simulink model "comprehensive_model_with_rocks_trial"  (R2019a)
settings: Solver=FixedStepAuto  StartTime=0.0  StopTime=15  FixedStep=0.001  RelTol=1e-3
PreLoadFcn:
  | load('tumbleweed_constants.mat')
values from neighbouring files (symbols this model uses):
  Ar = 0.785398163397    [tumbleweed_constants.mat]
  CD = 0.8    [tumbleweed_constants.mat]
  d = 0.65    [tumbleweed_constants.mat]
  g = 9.81    [tumbleweed_constants.mat]
  Ixx = 1.29    [tumbleweed_constants.mat]
  Iyy = 1.29    [tumbleweed_constants.mat]
  Izz = 1.29    [tumbleweed_constants.mat]
  m = 1    [tumbleweed_constants.mat]
  maxr = 0.45    [tumbleweed_constants.mat]
  mf = 14    [tumbleweed_constants.mat]
  minr = 0.2    [tumbleweed_constants.mat]
  mu0 = 0.02    [tumbleweed_constants.mat]
  muk = 0.5    [tumbleweed_constants.mat]
  must = 0.8    [tumbleweed_constants.mat]
  R = cylR*ones(size(Theta,1),size(Theta,2))    [d3_animate.m]    (also in tumbleweed_constants.mat = 0.5)
  rest_coeff = 0.6    [tumbleweed_constants.mat]
  rho = 1.2    [tumbleweed_constants.mat]
  ts = 0.5    [tumbleweed_constants.mat]
  v_thres = 0.0001    [tumbleweed_constants.mat]
  vmax = 0.2    [tumbleweed_constants.mat]
  YY = 50    [tumbleweed_constants.mat]
libraries: simulink x2
(part 3 of 9)

== matlab function comprehensive_model_with_rocks_trial/bouncing_model1/only_bounce/MATLAB Function1 ==
  data: t input; states input; constraint_flag output; r_AO output; par_diffs output; rock_cents input; rock_radi input; jAp input; surf_num input; R parameter; surf_numch output
function [constraint_flag, r_AO, par_diffs, surf_numch] = surf_constraint_check(t, states, rock_cents, rock_radi, jAp, surf_num, R)
if t == 3.431
    disp(t);
end
surf_numch = surf_num;
r_TO = [states(7);states(8);states(9)];
O_v_TO =[states(4);states(5);states(6)];
%change the surface equation in the dist_calc function and par_diffs_calc
point_on_surf = [0;0];
smallest_dist = 0;
rock_radi = rock_radi';
if t== 2.922
    disp(states)
end
[point_on_surf, smallest_dist] = dist_calc(r_TO);
z_c = surf_eq(point_on_surf(1),point_on_surf(2),r_TO);
r_AO = [point_on_surf;z_c];
par_diffs = par_diffs_calc(r_AO);
        fx = par_diffs(1,1); 
        fy = par_diffs(2,1);
        fz = par_diffs(3,1);
        kO = [0;0;1];
        iO = [1;0;0];
        jO = [0;1;0];

        if(abs(fx)<=1e-10 && abs(fy)<=1e-10)
            kA = kO;
            jA = jO;
            iA = iO;
            O_c_A = eye(3);
            A_c_O = eye(3);
            flag = 1;
        else
        kA = [fx;fy;fz]/norm([fx;fy;fz]);
        jA = cross(kO,kA)/norm(cross(kO,kA));
        flag = 1;
        if((jAp.')*(jA) < 0)
            jA = -jA;
            flag = 2;
        end
        iA = cross(jA,kA);
        A_c_O = [iA'*iO, iA'*jO, iA'*kO; jA'*iO, jA'*jO, jA'*kO; kA'*iO, kA'*jO, kA'*kO];
        O_c_A = transpose(A_c_O);
        end
O_v_TOa = A_c_O*O_v_TO;  

if norm(r_AO - r_TO) <= R + 0.00005 && O_v_TOa(3) <= 0
    constraint_flag = 1;
elseif norm(r_AO - r_TO) <= R - 0.002 && O_v_TOa(3) <= 0
    constraint_flag = 1;    
else 
    constraint_flag = 0;
end
rock_coll_flag = 0;
rock_ind = 0;

for i = 1:size(rock_cents,2) 
    if norm(r_TO - rock_cents(:,i)) <= rock_radi(1,i) + R + 0.001
        kR = (r_TO - rock_cents(:,i))/norm(r_TO -  rock_cents(:,i));   
       if(abs(kR(1))<=1e-10 && abs(kR(2))<=1e-10)
            kR = kO;
            jR = jO;
            iR = iO;
            O_c_R = eye(3);
            R_c_O = eye(3);
            flag = 1;
       else
        jR = cross(kO,kR)/norm(cross(kO,kR));
        flag = 1;
        if((jAp.')*(jR) < 0)
            jR = -jR;
            flag = 2;
        end
        iR = cross(jR,kR);
        R_c_O = [iR'*iO, iR'*jO, iR'*kO; jR'*iO, jR'*jO, jR'*kO; kR'*iO, kR'*jO, kR'*kO];
        O_c_R = transpose(R_c_O);
        end
    O_v_TOr = R_c_O*O_v_TO;  
        if O_v_TOr(3)<= 0
            rock_coll_flag = 1;
            rock_ind = i;
        end
    end
end
if (rock_coll_flag == 1 && constraint_flag == 0) 
kR = (r_TO - rock_cents(:,rock_ind))/norm(r_TO -  rock_cents(:,rock_ind));
point_on_rock = rock_cents(:,rock_ind) + rock_radi(1,rock_ind)*kR;
r_AO = point_on_rock;
par_diffs = rock_pardiffs_calc(point_on_rock, rock_cents(:,rock_ind));
surf_numch = rock_ind;
constraint_flag = 1;
elseif (rock_coll_flag == 1 && constraint_flag == 1)
kR = (r_TO - rock_cents(:,rock_ind))/norm(r_TO -  rock_cents(:,rock_ind));
point_on_rock = rock_cents(:,rock_ind) + rock_radi(1,rock_ind)*kR;
r_AO = point_on_rock;
par_diffs = rock_pardiffs_calc(point_on_rock, rock_cents(:,rock_ind));
surf_numch = 0;
elseif (rock_coll_flag == 0 && constraint_flag == 1)
    surf_numch = 0;
end
end




function rock_pardiffs = rock_pardiffs_calc(point_on_rock, rock_center)
r_RO = point_on_rock; x_c = r_RO(1); y_c = r_RO(2); z_c = r_RO(3);
r_CO = rock_center;
fx = 2*(x_c - r_CO(1,1));
fy = 2*(y_c - r_CO(2,1));
fz = 2*(z_c - r_CO(3,1));
fxx = 2;
fxy = 0;
fxz = 0;
fyy = 2;
fyz = 0;
fzz = 2;
fxxx = 0;
fxxy = 0;
fxxz = 0;
fxyy = 0;
fxyz = 0;
fxzz = 0;
fyyy = 0;
fyyz = 0;
fyzz = 0;
fzzz = 0;
rock_pardiffs = [fx;fy;fz;fxx;fxy;fxz;fyy;fyz;fzz;fxxx;fxxy;fxxz;fxyy;fxyz;fxzz;fyyy;fyyz;fyzz;fzzz];
end



function z_c = surf_eq(x_c, y_c, r_TO)
% if r_TO(3) >= 0
%     if x_c^2 - 2*y_c < 0
%         z_c = 0;
%     else
%     z_c = sqrt(x_c^2 - 2*y_c);
%     end
% else
%     if x_c^2 - 2*y_c < 0
%         z_c = 0;
%     else
%     z_c = -sqrt(x_c^2 - 2*y_c);
%     end
% end
z_c = 0;%(4*exp(-((x_c-5)^2 + (y_c)^2)/(6^2))-6*exp(-((x_c-5)^2 + (y_c)^2)/(4^2)));%(-1*exp(-((x_c - 10)^2 + (y_c - 10)^2)/2^2) -5*exp(-((x_c - 10)^2 + (y_c - 15)^2)/5^2) + 5*exp(-((x_c - 10)^2 + (y_c + 10)^2)/5^2) - 3*exp(-((x_c - 20)^2 + (y_c +5)^2)/4^2) - 5*exp(-((x_c - 40)^2 + (y_c -10)^2)/6^2));
end

function par_diffs = par_diffs_calc(r_AO)

x_c = r_AO(1);
y_c = r_AO(2);
z_c = r_AO(3);

fx = 0;%4*exp(- (x_c - 5)^2/36 - y_c^2/36)*(x_c/18 - 5/18) - 6*exp(- (x_c - 5)^2/16 - y_c^2/16)*(x_c/8 - 5/8);
fy = 0;%(2*y_c*exp(- (x_c - 5)^2/36 - y_c^2/36))/9 - (3*y_c*exp(- (x_c - 5)^2/16 - y_c^2/16))/4;
fz = 1;
fxx = 0;%(2*exp(- (x_c - 5)^2/36 - y_c^2/36))/9 - (3*exp(- (x_c - 5)^2/16 - y_c^2/16))/4 + 6*exp(- (x_c - 5)^2/16 - y_c^2/16)*(x_c/8 - 5/8)^2 - 4*exp(- (x_c - 5)^2/36 - y_c^2/36)*(x_c/18 - 5/18)^2;
fxy = 0;%(3*y_c*exp(- (x_c - 5)^2/16 - y_c^2/16)*(x_c/8 - 5/8))/4 - (2*y_c*exp(- (x_c - 5)^2/36 - y_c^2/36)*(x_c/18 - 5/18))/9;
fxz = 0;
fyy = 0;%(2*exp(- (x_c - 5)^2/36 - y_c^2/36))/9 - (3*exp(- (x_c - 5)^2/16 - y_c^2/16))/4 + (3*y_c^2*exp(- (x_c - 5)^2/16 - y_c^2/16))/32 - (y_c^2*exp(- (x_c - 5)^2/36 - y_c^2/36))/81;
fyz = 0;
fzz = 0;
fxxx = 0;%(3*exp(- (x_c - 5)^2/16 - y_c^2/16)*(x_c/8 - 5/8))/4 + 6*exp(- (x_c - 5)^2/16 - y_c^2/16)*(x_c/32 - 5/32) - (2*exp(- (x_c - 5)^2/36 - y_c^2/36)*(x_c/18 - 5/18))/9 - 4*exp(- (x_c - 5)^2/36 - y_c^2/36)*(x_c/162 - 5/162) - 6*exp(- (x_c - 5)^2/16 - y_c^2/16)*(x_c/8 - 5/8)^3 + 4*exp(- (x_c - 5)^2/36 - y_c^2/36)*(x_c/18 - 5/18)^3;
fxxy = 0;%(3*y_c*exp(- (x_c - 5)^2/16 - y_c^2/16))/32 - (y_c*exp(- (x_c - 5)^2/36 - y_c^2/36))/81 - (3*y_c*exp(- (x_c - 5)^2/16 - y_c^2/16)*(x_c/8 - 5/8)^2)/4 + (2*y_c*exp(- (x_c - 5)^2/36 - y_c^2/36)*(x_c/18 - 5/18)^2)/9;
fxxz = 0;
fxyy = 0;%(3*exp(- (x_c - 5)^2/16 - y_c^2/16)*(x_c/8 - 5/8))/4 - (2*exp(- (x_c - 5)^2/36 - y_c^2/36)*(x_c/18 - 5/18))/9 - (3*y_c^2*exp(- (x_c - 5)^2/16 - y_c^2/16)*(x_c/8 - 5/8))/32 + (y_c^2*exp(- (x_c - 5)^2/36 - y_c^2/36)*(x_c/18 - 5/18))/81;
fxyz = 0;
fxzz = 0;
fyyy = 0;%(9*y_c*exp(- (x_c - 5)^2/16 - y_c^2/16))/32 - (y_c*exp(- (x_c - 5)^2/36 - y_c^2/36))/27 - (3*y_c^3*exp(- (x_c - 5)^2/16 - y_c^2/16))/256 + (y_c^3*exp(- (x_c - 5)^2/36 - y_c^2/36))/1458;
fyyz = 0;
fyzz = 0;
fzzz = 0;


% fx = -x_c;
% fy = 1;
% fz = z_c;
% fxx = -1;
% fxy = 0;
% fxz = 0;
% fyy = 0;
% fyz = 0;
% fzz = 1;
% fxxx = 0;
% fxxy = 0;
% fxxz = 0;
% fxyy = 0;
% fxyz = 0;
% fxzz = 0;
% fyyy = 0;
% fyyz = 0;
% fyzz = 0;
% fzzz = 0;
% 


par_diffs = [fx;fy;fz;fxx;fxy;fxz;fyy;fyz;fzz;fxxx;fxxy;fxxz;fxyy;fxyz;fxzz;fyyy;fyyz;fyzz;fzzz];
end

== matlab function comprehensive_model_with_rocks_trial/Subsystem1/MATLAB Function ==
  data: t input; y output size=3; ydot output size=3; states input; hit input; hit output; R parameter; y_new input; y_new output; err input; cum_err input; err output; cum_err output; rand_num input; stop_flag output
function [y, ydot,hit, y_new,err,cum_err,stop_flag] = reference_trajectory_generator(t,states,hit,R,y_new,err,cum_err,rand_num)

% xr = y_new;
% yr = 30*sin(xr/(30*pi));
% zr = R;
% 
% if abs(states(7) - xr) <= 0.5    
% xr = xr + 5;
% y_new = xr;
% cum_err = cum_err + abs(states(8) - yr);
% err = abs(states(8) - yr);
% yr = 30*sin(xr/(30*pi));
% zr = R; 
% end
% 
% xr_dot = 0;
% yr_dot = 0;
% zr_dot = 0;

if hit == 0
 xr = 800;
 yr = 1000;
 zr = R;
        
 
xr_dot = 0;
yr_dot = 0;
zr_dot = 0;
elseif hit == 1
 xr = states(7);
 yr = y_new(2);
 zr = R;
        
 
xr_dot = 0;
yr_dot = 0;
zr_dot = 0;
% elseif hit == 2
%      xr = 150;
%  yr = -40;
%  zr = R;
%         
% % 
% xr_dot = 0;
% yr_dot = 0;
% zr_dot = 0;
% elseif hit == 3
% xr = 200;
%  yr = -10;
%  zr = R;
%         
% 
% xr_dot = 0;
% yr_dot = 0;
% zr_dot = 0;
else
 xr = states(7);
 yr = y_new(2);
 zr = R;


xr_dot = 0;
yr_dot = 0;
zr_dot = 0;
end
% 
if hit == 0 && abs(states(7) - xr )<=0.5
    hit = 1;
    y_new = [states(7);states(8)];
% elseif hit == 1 && abs(states(7) -xr)<=0.5
%     hit = 2;
% elseif hit == 2 && abs(states(8) - yr)<=0.5
%     hit = 3;
% elseif hit == 3 && abs(states(8) - yr)<=0.5
%     hit = 4;
else
    hit = hit;
end
% 
% xr = 0.1*t;
% yr = 15*sin(0.1/4*t);
% zr = R;
% 
% xr_dot = 0.1;
% yr_dot = 15*cos(0.1/4*t)*(0.1/4);
% zr_dot = 0;
% if abs(xr - 10) <= 0.5
%     xr = states(7);
%     yr = 1000;
%     zr = R;
% else
% xr = states(7);
% yr = 1000;
% zr = R;
% end
% 
% xr_dot = 0;
% yr_dot = 0;
% zr_dot =0;
% xr = 30*cos(0.062/3*t);
% yr = 30*sin(0.062/3*t);
% zr = R;
% xr_dot = -30*sin(0.062/3*t)*(0.062/3);
% yr_dot = 30*cos(0.062/3*t)*(0.062/3);
% zr_dot = 0;

% 
% if abs(states(7) - y_new(1))<=0.5
% cum_err = abs(states(8) - y_new(2));
% y_new(1) = y_new(1) + 50;    
% if mod(((states(7) - rem(states(7),500))/500),2) == 0 
% y_new(2) = states(8) + 15*rand_num;
% else
%     y_new(2) = states(8) - 15*rand_num;
% end
% err = [states(7);states(8)];
% 
% 
% end
% xr = y_new(1);
% yr = y_new(2);
% zr = R;
% 
% xr_dot = 0;
% yr_dot = 0;
% zr_dot = 0;

if abs(states(7) - y_new(1))<=1
    y_new(1) = y_new(1) + 10;   
    y_new(2) = 50*sin(y_new(1)*2*pi/750);
    err = [states(7);states(8)];
end

xr = y_new(1);
yr = y_new(2);
zr = R;
xr_dot = 0;
yr_dot = 0;
zr_dot = 0;

if states(7) > 750
    stop_flag = 1;
else
    stop_flag = 0;
end
y = [xr;yr;zr];
ydot = [xr_dot; yr_dot; zr_dot];
 

end

== matlab function comprehensive_model_with_rocks_trial/command filter based backstepper/Subsystem1/MATLAB Function ==
  data: u input; f3_u output size=3; u_dot input; u_ddot input; states input; FW input; v_thres parameter; d parameter; R parameter; mu0 parameter; mf parameter; m parameter; Izz parameter; Iyy parameter; Ixx parameter; g parameter
function f3_u = f3u_calculator(u,u_dot,u_ddot,states,FW,v_thres, d, R, mu0, mf, m, Izz, Iyy, Ixx, g)
I_T = [Ixx,0,0;0,Iyy,0;0,0,Izz];
r_m1T = [u(1);0;0];             T_v_m1T = [u_dot(1);0;0]; T_a_m1T = [u_ddot(1);0;0];
r_m2T = [-(d - u(1));0;0];      T_v_m2T = [u_dot(1);0;0]; T_a_m2T = [u_ddot(1);0;0];
r_m3T = [0;u(2);0];             T_v_m3T = [0;u_dot(2);0]; T_a_m3T = [0;u_ddot(2);0];
r_m4T = [0;-(d - u(2));0];      T_v_m4T = [0;u_dot(2);0]; T_a_m4T = [0;u_ddot(2);0];
r_m5T = [0;0;u(3)];             T_v_m5T = [0;0;u_dot(3)]; T_a_m5T = [0;0;u_ddot(3)];
r_m6T = [0;0;-(d - u(3))];      T_v_m6T = [0;0;u_dot(3)]; T_a_m6T = [0;0;u_ddot(3)];
r_CMT = m*(r_m1T + r_m2T + r_m3T + r_m4T + r_m5T + r_m6T)/(6*m+mf);
T_v_CMT = m*(T_v_m1T + T_v_m2T + T_v_m3T + T_v_m4T + T_v_m5T + T_v_m6T)/(6*m+mf);
T_a_CMT = m*(T_a_m1T + T_a_m2T + T_a_m3T + T_a_m4T + T_a_m5T + T_a_m6T)/(6*m+mf);
r_CMTx = Vx(r_CMT);r_m1Tx = Vx(r_m1T);r_m2Tx = Vx(r_m2T);r_m3Tx = Vx(r_m3T);
r_m4Tx = Vx(r_m4T);r_m5Tx = Vx(r_m5T);r_m6Tx = Vx(r_m6T);
q0 = states(10);q1=states(11);q2=states(12);q3=states(13);
T_c_O = [q0^2 + q1^2 - q2^2 - q3^2, 2*(q1*q2 + q0*q3), 2*(q1*q3 - q0*q2);...
       2*(q1*q2 - q0*q3), q0^2 - q1^2 + q2^2 - q3^2, 2*(q2*q3 + q0*q1);...
       2*(q1*q3 + q0*q2), 2*(q2*q3 - q0*q1), q0^2 - q1^2 - q2^2 + q3^2];
O_c_T = transpose(T_c_O);  
r_PT = [0;0;-R];
r_PTx = Vx([0;0;-R]);
O_w_T = [states(1);states(2);states(3)]; O_w_Tx =Vx(O_w_T);

O_vel_TO = Vx(O_c_T*O_w_T)*[0;0;R];
u_TO = O_vel_TO(1);
v_TO = O_vel_TO(2);

murr = mu0*tanh((u_TO^2 + v_TO^2)/v_thres); 
roll_rest_coeff = [1,0,-murr*u_TO/sqrt(u_TO^2 + v_TO^2);0,1,-murr*v_TO/sqrt(u_TO^2 + v_TO^2);0,0,1];
FG = [0;0;-(mf+6*m)*g];
FR  = -murr*norm(FG)/sqrt(u_TO^2 + v_TO^2)*[u_TO; v_TO; 0];

f3_u = zeros(3,1);
Amat = I_T + (mf + 6*m)*r_CMTx*T_c_O*r_PTx*O_c_T - m*r_m1Tx*r_m1Tx - m*r_m2Tx*r_m2Tx...
       - m*r_m3Tx*r_m3Tx - m*r_m4Tx*r_m4Tx - m*r_m5Tx*r_m5Tx - m*r_m6Tx*r_m6Tx...
       - (mf + 6*m)*Vx(T_c_O*r_PT)*Vx(T_c_O*r_PT) + (mf + 6*m)*Vx(T_c_O*r_PT)*r_CMTx;
  %some mistakes here. check again 
Bvec = -cross(O_w_T,I_T*O_w_T) - m*cross(r_m1T,2*O_w_Tx*T_v_m1T + O_w_Tx*O_w_Tx*r_m1T)...
       - m*r_m2Tx*(T_a_m2T + 2*O_w_Tx*T_v_m2T + O_w_Tx*O_w_Tx*r_m2T)...
       - m*r_m3Tx*(T_a_m3T + 2*O_w_Tx*T_v_m3T + O_w_Tx*O_w_Tx*r_m3T)...
       - m*r_m4Tx*(T_a_m4T + 2*O_w_Tx*T_v_m4T + O_w_Tx*O_w_Tx*r_m4T)...
       - m*r_m5Tx*(T_a_m5T + 2*O_w_Tx*T_v_m5T + O_w_Tx*O_w_Tx*r_m5T)...
       - m*r_m6Tx*(T_a_m6T + 2*O_w_Tx*T_v_m6T + O_w_Tx*O_w_Tx*r_m6T)...
       + r_CMTx*T_c_O*FG + (mf + 6*m)*cross(T_c_O*r_PT, T_a_CMT + ...
         2*O_w_Tx*T_v_CMT + O_w_Tx*O_w_Tx*r_CMT) - T_c_O*cross(r_PT, FG) ...
         - T_c_O*cross(r_PT, FW);%- T_c_O*cross(r_PT, FR);
f3_u = inv(Amat)*Bvec;
end

== matlab function comprehensive_model_with_rocks_trial/bouncing_model/MATLAB Function ==
  data: t input; states_inair input; states output; states_onsurface input; FW_inair input; FW_onsurface input; inair_flag input; FW output; inactive_time input; inactive_time output; stop_flag output
function [states, FW, inactive_time, stop_flag] = merger(t,states_inair, states_onsurface, FW_inair, FW_onsurface, inair_flag, inactive_time)
if inair_flag > 0
    states = states_inair;
    FW = FW_inair;
    if norm(states) == 0
        states = states_onsurface;
        FW = FW_onsurface;
    end
else
    states = states_onsurface;
    FW = FW_onsurface;
    if norm(states) == 0
        states = states_inair;
         FW = FW_inair;
    end
    if mod(t,0.1) == 0
        if norm(states(4:6)) <= 0.005
            inactive_time = inactive_time + 0.1;
        else
            inactive_time = 0;
        end
    end
end

if inactive_time >= 50
    stop_flag = 1;
else
    stop_flag = 0;
end

end

== matlab function comprehensive_model_with_rocks_trial/bouncing_model/onsurface_model/MATLAB Function11 ==
  data: states input; wv input; FW output; CD parameter; rho parameter; Ar parameter
function FW = wind_force_calc(states,wv, CD, rho, Ar)
O_v_wO = [wv;0;0];
O_v_TO = [states(4);states(5);states(6)];
O_v_Tw = O_v_TO - O_v_wO;
FW = -0.5*CD*rho*Ar*norm(O_v_Tw)^2*O_v_Tw/norm(O_v_Tw);
%FW = zeros(3,1);
end

== matlab function comprehensive_model_with_rocks_trial/bouncing_model/onsurface_model/MATLAB Function2 ==
  data: r_AO input; r_AO0 input; roll_reset_flag input; par_diffs output; surf_num input; rock_cents input
function par_diffs = par_diffs_calc(r_AO, r_AO0, roll_reset_flag, surf_num, rock_cents)
if roll_reset_flag == 1
    r_AO = r_AO0;
end
x_c = r_AO(1);
y_c = r_AO(2);
z_c = r_AO(3);

if surf_num == 0
fx = 0;%4*exp(- (x_c - 5)^2/36 - y_c^2/36)*(x_c/18 - 5/18) - 6*exp(- (x_c - 5)^2/16 - y_c^2/16)*(x_c/8 - 5/8);
fy = 0;%(2*y_c*exp(- (x_c - 5)^2/36 - y_c^2/36))/9 - (3*y_c*exp(- (x_c - 5)^2/16 - y_c^2/16))/4;
fz = 1;
fxx = 0;%(2*exp(- (x_c - 5)^2/36 - y_c^2/36))/9 - (3*exp(- (x_c - 5)^2/16 - y_c^2/16))/4 + 6*exp(- (x_c - 5)^2/16 - y_c^2/16)*(x_c/8 - 5/8)^2 - 4*exp(- (x_c - 5)^2/36 - y_c^2/36)*(x_c/18 - 5/18)^2;
fxy = 0;%(3*y_c*exp(- (x_c - 5)^2/16 - y_c^2/16)*(x_c/8 - 5/8))/4 - (2*y_c*exp(- (x_c - 5)^2/36 - y_c^2/36)*(x_c/18 - 5/18))/9;
fxz = 0;
fyy = 0;%(2*exp(- (x_c - 5)^2/36 - y_c^2/36))/9 - (3*exp(- (x_c - 5)^2/16 - y_c^2/16))/4 + (3*y_c^2*exp(- (x_c - 5)^2/16 - y_c^2/16))/32 - (y_c^2*exp(- (x_c - 5)^2/36 - y_c^2/36))/81;
fyz = 0;
fzz = 0;
fxxx = 0;%(3*exp(- (x_c - 5)^2/16 - y_c^2/16)*(x_c/8 - 5/8))/4 + 6*exp(- (x_c - 5)^2/16 - y_c^2/16)*(x_c/32 - 5/32) - (2*exp(- (x_c - 5)^2/36 - y_c^2/36)*(x_c/18 - 5/18))/9 - 4*exp(- (x_c - 5)^2/36 - y_c^2/36)*(x_c/162 - 5/162) - 6*exp(- (x_c - 5)^2/16 - y_c^2/16)*(x_c/8 - 5/8)^3 + 4*exp(- (x_c - 5)^2/36 - y_c^2/36)*(x_c/18 - 5/18)^3;
fxxy = 0;%(3*y_c*exp(- (x_c - 5)^2/16 - y_c^2/16))/32 - (y_c*exp(- (x_c - 5)^2/36 - y_c^2/36))/81 - (3*y_c*exp(- (x_c - 5)^2/16 - y_c^2/16)*(x_c/8 - 5/8)^2)/4 + (2*y_c*exp(- (x_c - 5)^2/36 - y_c^2/36)*(x_c/18 - 5/18)^2)/9;
fxxz = 0;
fxyy = 0;%(3*exp(- (x_c - 5)^2/16 - y_c^2/16)*(x_c/8 - 5/8))/4 - (2*exp(- (x_c - 5)^2/36 - y_c^2/36)*(x_c/18 - 5/18))/9 - (3*y_c^2*exp(- (x_c - 5)^2/16 - y_c^2/16)*(x_c/8 - 5/8))/32 + (y_c^2*exp(- (x_c - 5)^2/36 - y_c^2/36)*(x_c/18 - 5/18))/81;
fxyz = 0;
fxzz = 0;
fyyy = 0;%(9*y_c*exp(- (x_c - 5)^2/16 - y_c^2/16))/32 - (y_c*exp(- (x_c - 5)^2/36 - y_c^2/36))/27 - (3*y_c^3*exp(- (x_c - 5)^2/16 - y_c^2/16))/256 + (y_c^3*exp(- (x_c - 5)^2/36 - y_c^2/36))/1458;
fyyz = 0;
fyzz = 0;
fzzz = 0;
else 

r_CO = rock_cents(:,surf_num).';
fx = 2*(x_c - r_CO(1));
fy = 2*(y_c - r_CO(2));
fz = 2*(z_c - r_CO(3));
fxx = 2;
fxy = 0;
fxz = 0;
fyy = 2;
fyz = 0;
fzz = 2;
fxxx = 0;
fxxy = 0;
fxxz = 0;
fxyy = 0;
fxyz = 0;
fxzz = 0;
fyyy = 0;
fyyz = 0;
fyzz = 0;
fzzz = 0;
end


% fx = -x_c;
% fy = 1;
% fz = z_c;
% fxx = -1;
% fxy = 0;
% fxz = 0;
% fyy = 0;
% fyz = 0;
% fzz = 1;
% fxxx = 0;
% fxxy = 0;
% fxxz = 0;
% fxyy = 0;
% fxyz = 0;
% fxzz = 0;
% fyyy = 0;
% fyyz = 0;
% fyzz = 0;
% fzzz = 0;
par_diffs = [fx;fy;fz;fxx;fxy;fxz;fyy;fyz;fzz;fxxx;fxxy;fxxz;fxyy;fxyz;fxzz;fyyy;fyyz;fyzz;fzzz];
end

== matlab function comprehensive_model_with_rocks_trial/bouncing_model/onsurface_model/MATLAB Function3 ==
  data: O_c_A input; states input; FN input; inair_flag output; FN output
function [inair_flag,FN] = inair_flag_set(O_c_A,states,FN)
O_v_TO = states(4:6,1);
A_c_O = O_c_A';
O_v_TOa = A_c_O*O_v_TO;
if FN < 0 || O_v_TOa(3) > 0.0001
    inair_flag = 1;
    FN = -1;
elseif O_v_TOa(3) < -0.008
    inair_flag = 1;
    FN = 100;
else
    inair_flag = 0;
end
end

== matlab function comprehensive_model_with_rocks_trial/bouncing_model/only_bounce/MATLAB Function2 ==
  data: t input; states input; u input; r_AO input; constraint_flag input; states output; roll_reset_flag output; FN input; inair_reset_flag output; par_diffs input; jAp input; surf_numch input; surf_nump input; rest_coeff parameter; m parameter; mf parameter; Ixx parameter; R parameter; jA output; must parameter; muk parameter; FN output; surf_num output; Iyy parameter; Izz parameter
function [states, roll_reset_flag, inair_reset_flag, jA, FN, surf_num] = collision_state_set(t,states, u,r_AO, constraint_flag, FN, par_diffs, jAp, surf_numch, surf_nump, rest_coeff, m, mf, Ixx, R, must, muk, Iyy, Izz)
%u1 u2 u3 u4 u5 u6 S1 S2 S3
surf_num = surf_nump;
roll_reset_flag = 0;
inair_reset_flag = 0;
O_w_T = [states(1);states(2);states(3)];
O_v_TO = [states(4);states(5);states(6)];
r_TO = [states(7);states(8);states(9)];
q = [states(10);states(11);states(12);states(13)];
q0 = q(1); q1 = q(2); q2 = q(3); q3 = q(4);

        fx = par_diffs(1,1); 
        fy = par_diffs(2,1);
        fz = par_diffs(3,1);
        kO = [0;0;1];
        iO = [1;0;0];
        jO = [0;1;0];

        if(abs(fx)<=1e-10 && abs(fy)<=1e-10)
            kA = kO;
            jA = jO;
            iA = iO;
            O_c_A = eye(3);
            A_c_O = eye(3);
            flag = 1;
        else
        kA = [fx;fy;fz]/norm([fx;fy;fz]);
        jA = cross(kO,kA)/norm(cross(kO,kA));
        flag = 1;
        if((jAp.')*(jA) < 0)
            jA = -jA;
            flag = 2;
        end
        iA = cross(jA,kA);
        A_c_O = [iA'*iO, iA'*jO, iA'*kO; jA'*iO, jA'*jO, jA'*kO; kA'*iO, kA'*jO, kA'*kO];
        O_c_A = transpose(A_c_O);
        end
O_v_TOa = A_c_O*O_v_TO;        
        
if mod(t,0.001) == 0
if constraint_flag == 0
    inair_flag = true;
 elseif constraint_flag == 1 && FN == 0
             inair_flag = false;
            roll_reset_flag = 1;
            r_TO = r_AO + R*kA;
            surf_num = surf_numch;
elseif constraint_flag == 1 && O_v_TOa(3) >= 0.0001
    inair_flag = true;    
else 
 %%collision response
     
        T_c_O = [q0^2 + q1^2 - q2^2 - q3^2, 2*(q1*q2 + q0*q3), 2*(q1*q3 - q0*q2);...
        2*(q1*q2 - q0*q3), q0^2 - q1^2 + q2^2 - q3^2, 2*(q2*q3 + q0*q1);...
        2*(q1*q3 + q0*q2), 2*(q2*q3 - q0*q1), q0^2 - q1^2 - q2^2 + q3^2];
        O_c_T = T_c_O.';
       
        
        
        T_c_A = T_c_O*O_c_A;
        A_c_T = T_c_A.';
        
        
        l1 = u(1); l2 = u(2); l3 = u(3); l4 = u(4); l5 = u(5); l6 = u(6);
        L33 = Ixx + m*(l3^2 + l4^2 + l5^2 + l6^2);
        L11 = Iyy + m*(l1^2 + l2^2 + l5^2 + l6^2);
        L22 = Izz + m*(l3^2 + l4^2 + l1^2 + l2^2);
        L = A_c_T*[L33,0,0;0,L11,0;0,0,L22]*T_c_A;
        L11 = L(2,2);
        L22 = L(3,3);
        L33 = L(1,1);
        
        mT = mf +6*m;

        w = A_c_T*(O_w_T);
        v = A_c_O*O_v_TO;

        u3 = w(1,1);
        u2 = w(3,1);
        u1 = w(2,1);

        u6 = v(1,1);
        u5 = v(3,1);
        u4 = v(2,1);


        u5_n = -rest_coeff*u5;  
        if abs(u5_n) <= 0.005 %&& FN > 0
            u5_n = 0;
            inair_flag = false;
            roll_reset_flag = 1;
            surf_num = surf_numch;
            r_TO = r_AO + R*kA;
%         elseif abs(u5_n) <= 0.005 && FN < 0
%             u5_n = 0;
%             inair_flag = true;
%             r_TO = r_AO + R*kA;   
        else
            inair_flag = true;
            inair_reset_flag = 1;
             r_TO = r_AO + R*kA;
             FN = 100;
        end
        u2_n = u2;
        u3_n = (L33*u3 - mT*R*u4)/(mT*R^2 + L33);
        u4_n = -R*u3_n;
        u1_n = (L11*u1 + mT*R*u6)/(mT*R^2 + L11);
        u6_n = R*u1_n;
        S1 = mT*(u4_n - u4);
        S2 = mT*(u5_n - u5);
        S3 = mT*(u6_n - u6);

        if ~(sqrt(S1^2 + S3^2) < must*norm(S2))
            alpha = u4 + R*u3;
            gamma = u6 - R*u1;
            k1 = 1/mT + R^2/L11;
            k3 = 1/mT + R^2/L33;
            
            if abs(alpha) > 0
                S1 = S1solve(S2, muk,alpha, gamma, k1, k3); 
                S3 = gamma*S1/(alpha + (k3 - k1)*S1);
                u1_n = u1 - R*S3/L11;
                u3_n = u3 + R*S1/L33;
                u4_n = u4 + S1/mT;
                u6_n = u6 + S3/mT;
            else 
                S3 = S1solve(S2, muk, gamma, alpha, k3, k1);
                S1 = alpha*S3/(gamma + (k1 - k3)*S3);
                u1_n = u1 - R*S3/L11;
                u3_n = u3 + R*S1/L33;
                u4_n = u4 + S1/mT;
                u6_n = u6 + S3/mT;
            end
            
        end

        O_w_T = T_c_A*[u3_n;u1_n;u2_n];
        O_v_TO = O_c_A*[u6_n; u4_n; u5_n];
end
else
    if  constraint_flag == 0
        inair_flag = true;
    else
        inair_flag = false;
    end
end

states = [O_w_T;O_v_TO;r_TO;q];
end

== matlab function comprehensive_model_with_rocks_trial/bouncing_model/only_bounce/MATLAB Function1 ==
  data: t input; states input; constraint_flag output; r_AO output; par_diffs output; rock_cents input; rock_radi input; jAp input; surf_num input; R parameter; surf_numch output
function [constraint_flag, r_AO, par_diffs, surf_numch] = surf_constraint_check(t, states, rock_cents, rock_radi, jAp, surf_num, R)
surf_numch = surf_num;
r_TO = [states(7);states(8);states(9)];
O_v_TO =[states(4);states(5);states(6)];
%change the surface equation in the dist_calc function and par_diffs_calc
point_on_surf = [0;0];
smallest_dist = 0;
rock_radi = rock_radi';
 [point_on_surf, smallest_dist] = dist_calc(r_TO);
% point_on_surf = [r_TO(1);r_TO(2)];
% smallest_dist = r_TO(3);
z_c = surf_eq(point_on_surf(1),point_on_surf(2),r_TO);
r_AO = [point_on_surf;z_c];
par_diffs = par_diffs_calc(r_AO);
        fx = par_diffs(1,1); 
        fy = par_diffs(2,1);
        fz = par_diffs(3,1);
        kO = [0;0;1];
        iO = [1;0;0];
        jO = [0;1;0];

        if(abs(fx)<=1e-10 && abs(fy)<=1e-10)
            kA = kO;
            jA = jO;
            iA = iO;
            O_c_A = eye(3);
            A_c_O = eye(3);
            flag = 1;
        else
        kA = [fx;fy;fz]/norm([fx;fy;fz]);
        jA = cross(kO,kA)/norm(cross(kO,kA));
        flag = 1;
        if((jAp.')*(jA) < 0)
            jA = -jA;
            flag = 2;
        end
        iA = cross(jA,kA);
        A_c_O = [iA'*iO, iA'*jO, iA'*kO; jA'*iO, jA'*jO, jA'*kO; kA'*iO, kA'*jO, kA'*kO];
        O_c_A = transpose(A_c_O);
        end
O_v_TOa = A_c_O*O_v_TO;  

if norm(r_AO - r_TO) <= R + 0.00005 && O_v_TOa(3) <= 0
    constraint_flag = 1;
elseif norm(r_AO - r_TO) <= R - 0.002 && O_v_TOa(3) <= 0
    constraint_flag = 1;    
else 
    constraint_flag = 0;
end
rock_coll_flag = 0;
rock_ind = 0;

for i = 1:size(rock_cents,2) 
    if norm(r_TO - rock_cents(:,i)) <= rock_radi(1,i) + R + 0.001
        kR = (r_TO - rock_cents(:,i))/norm(r_TO -  rock_cents(:,i));   
       if(abs(kR(1))<=1e-10 && abs(kR(2))<=1e-10)
            kR = kO;
            jR = jO;
            iR = iO;
            O_c_R = eye(3);
            R_c_O = eye(3);
            flag = 1;
       else
        jR = cross(kO,kR)/norm(cross(kO,kR));
        flag = 1;
        if((jAp.')*(jR) < 0)
            jR = -jR;
            flag = 2;
        end
        iR = cross(jR,kR);
        R_c_O = [iR'*iO, iR'*jO, iR'*kO; jR'*iO, jR'*jO, jR'*kO; kR'*iO, kR'*jO, kR'*kO];
        O_c_R = transpose(R_c_O);
        end
    O_v_TOr = R_c_O*O_v_TO;  
        if O_v_TOr(3)<= 0
            rock_coll_flag = 1;
            rock_ind = i;
        end
    end
end
if (rock_coll_flag == 1 && constraint_flag == 0) 
kR = (r_TO - rock_cents(:,rock_ind))/norm(r_TO -  rock_cents(:,rock_ind));
point_on_rock = rock_cents(:,rock_ind) + rock_radi(1,rock_ind)*kR;
r_AO = point_on_rock;
par_diffs = rock_pardiffs_calc(point_on_rock, rock_cents(:,rock_ind));
surf_numch = rock_ind;
constraint_flag = 1;
elseif (rock_coll_flag == 1 && constraint_flag == 1)
kR = (r_TO - rock_cents(:,rock_ind))/norm(r_TO -  rock_cents(:,rock_ind));
point_on_rock = rock_cents(:,rock_ind) + rock_radi(1,rock_ind)*kR;
r_AO = point_on_rock;
par_diffs = rock_pardiffs_calc(point_on_rock, rock_cents(:,rock_ind));
surf_numch = 0;
elseif (rock_coll_flag == 0 && constraint_flag == 1)
    surf_numch = 0;
end
end




function rock_pardiffs = rock_pardiffs_calc(point_on_rock, rock_center)
r_RO = point_on_rock; x_c = r_RO(1); y_c = r_RO(2); z_c = r_RO(3);
r_CO = rock_center;
fx = 2*(x_c - r_CO(1,1));
fy = 2*(y_c - r_CO(2,1));
fz = 2*(z_c - r_CO(3,1));
fxx = 2;
fxy = 0;
fxz = 0;
fyy = 2;
fyz = 0;
fzz = 2;
fxxx = 0;
fxxy = 0;
fxxz = 0;
fxyy = 0;
fxyz = 0;
fxzz = 0;
fyyy = 0;
fyyz = 0;
fyzz = 0;
fzzz = 0;
rock_pardiffs = [fx;fy;fz;fxx;fxy;fxz;fyy;fyz;fzz;fxxx;fxxy;fxxz;fxyy;fxyz;fxzz;fyyy;fyyz;fyzz;fzzz];
end



function z_c = surf_eq(x_c, y_c, r_TO)
% if r_TO(3) >= 0
%     if x_c^2 - 2*y_c < 0
%         z_c = 0;
%     else
%     z_c = sqrt(x_c^2 - 2*y_c);
%     end
% else
%     if x_c^2 - 2*y_c < 0
%         z_c = 0;
%     else
%     z_c = -sqrt(x_c^2 - 2*y_c);
%     end
% end
z_c = 0;%(4*exp(-((x_c-5)^2 + (y_c)^2)/(6^2))-6*exp(-((x_c-5)^2 + (y_c)^2)/(4^2)));%(-1*exp(-((x_c - 10)^2 + (y_c - 10)^2)/2^2) -5*exp(-((x_c - 10)^2 + (y_c - 15)^2)/5^2) + 5*exp(-((x_c - 10)^2 + (y_c + 10)^2)/5^2) - 3*exp(-((x_c - 20)^2 + (y_c +5)^2)/4^2) - 5*exp(-((x_c - 40)^2 + (y_c -10)^2)/6^2));
end

function par_diffs = par_diffs_calc(r_AO)

x_c = r_AO(1);
y_c = r_AO(2);
z_c = r_AO(3);

fx = 0;%4*exp(- (x_c - 5)^2/36 - y_c^2/36)*(x_c/18 - 5/18) - 6*exp(- (x_c - 5)^2/16 - y_c^2/16)*(x_c/8 - 5/8);
fy = 0;%(2*y_c*exp(- (x_c - 5)^2/36 - y_c^2/36))/9 - (3*y_c*exp(- (x_c - 5)^2/16 - y_c^2/16))/4;
fz = 1;
fxx = 0;%(2*exp(- (x_c - 5)^2/36 - y_c^2/36))/9 - (3*exp(- (x_c - 5)^2/16 - y_c^2/16))/4 + 6*exp(- (x_c - 5)^2/16 - y_c^2/16)*(x_c/8 - 5/8)^2 - 4*exp(- (x_c - 5)^2/36 - y_c^2/36)*(x_c/18 - 5/18)^2;
fxy = 0;%(3*y_c*exp(- (x_c - 5)^2/16 - y_c^2/16)*(x_c/8 - 5/8))/4 - (2*y_c*exp(- (x_c - 5)^2/36 - y_c^2/36)*(x_c/18 - 5/18))/9;
fxz = 0;
fyy = 0;%(2*exp(- (x_c - 5)^2/36 - y_c^2/36))/9 - (3*exp(- (x_c - 5)^2/16 - y_c^2/16))/4 + (3*y_c^2*exp(- (x_c - 5)^2/16 - y_c^2/16))/32 - (y_c^2*exp(- (x_c - 5)^2/36 - y_c^2/36))/81;
fyz = 0;
fzz = 0;
fxxx = 0;%(3*exp(- (x_c - 5)^2/16 - y_c^2/16)*(x_c/8 - 5/8))/4 + 6*exp(- (x_c - 5)^2/16 - y_c^2/16)*(x_c/32 - 5/32) - (2*exp(- (x_c - 5)^2/36 - y_c^2/36)*(x_c/18 - 5/18))/9 - 4*exp(- (x_c - 5)^2/36 - y_c^2/36)*(x_c/162 - 5/162) - 6*exp(- (x_c - 5)^2/16 - y_c^2/16)*(x_c/8 - 5/8)^3 + 4*exp(- (x_c - 5)^2/36 - y_c^2/36)*(x_c/18 - 5/18)^3;
fxxy = 0;%(3*y_c*exp(- (x_c - 5)^2/16 - y_c^2/16))/32 - (y_c*exp(- (x_c - 5)^2/36 - y_c^2/36))/81 - (3*y_c*exp(- (x_c - 5)^2/16 - y_c^2/16)*(x_c/8 - 5/8)^2)/4 + (2*y_c*exp(- (x_c - 5)^2/36 - y_c^2/36)*(x_c/18 - 5/18)^2)/9;
fxxz = 0;
fxyy =0;%(3*exp(- (x_c - 5)^2/16 - y_c^2/16)*(x_c/8 - 5/8))/4 - (2*exp(- (x_c - 5)^2/36 - y_c^2/36)*(x_c/18 - 5/18))/9 - (3*y_c^2*exp(- (x_c - 5)^2/16 - y_c^2/16)*(x_c/8 - 5/8))/32 + (y_c^2*exp(- (x_c - 5)^2/36 - y_c^2/36)*(x_c/18 - 5/18))/81;
fxyz = 0;
fxzz = 0;
fyyy =0;%(9*y_c*exp(- (x_c - 5)^2/16 - y_c^2/16))/32 - (y_c*exp(- (x_c - 5)^2/36 - y_c^2/36))/27 - (3*y_c^3*exp(- (x_c - 5)^2/16 - y_c^2/16))/256 + (y_c^3*exp(- (x_c - 5)^2/36 - y_c^2/36))/1458;
fyyz = 0;
fyzz = 0;
fzzz = 0;


% fx = -x_c;
% fy = 1;
% fz = z_c;
% fxx = -1;
% fxy = 0;
% fxz = 0;
% fyy = 0;
% fyz = 0;
% fzz = 1;
% fxxx = 0;
% fxxy = 0;
% fxxz = 0;
% fxyy = 0;
% fxyz = 0;
% fxzz = 0;
% fyyy = 0;
% fyyz = 0;
% fyzz = 0;
% fzzz = 0;
% 


par_diffs = [fx;fy;fz;fxx;fxy;fxz;fyy;fyz;fzz;fxxx;fxxy;fxxz;fxyy;fxyz;fxzz;fyyy;fyyz;fyzz;fzzz];
end

== matlab function comprehensive_model_with_rocks_trial/bouncing_model/only_bounce/MATLAB Function11 ==
  data: states input; FW output; CD parameter; rho parameter; Ar parameter; wx input
function FW = wind_force_calc(states, CD, rho, Ar,wx)
O_v_wO = [wx;0;0];
O_v_TO = [states(4);states(5);states(6)];
O_v_Tw = O_v_TO - O_v_wO;
FW = -0.5*CD*rho*Ar*norm(O_v_Tw)^2*O_v_Tw/norm(O_v_Tw);
%FW = zeros(3,1);
end

== matlab function comprehensive_model_with_rocks_trial/bouncing_model1/only_bounce/MATLAB Function11 ==
  data: states input; wx input; FW output; CD parameter; rho parameter; Ar parameter
function FW = wind_force_calc(states, wx,CD, rho, Ar)
O_v_wO = [wx;0;0];
O_v_TO = [states(4);states(5);states(6)];
O_v_Tw = O_v_TO - O_v_wO;
FW = -0.5*CD*rho*Ar*norm(O_v_Tw)^2*O_v_Tw/norm(O_v_Tw);
%FW = zeros(3,1);
end

== matlab function comprehensive_model_with_rocks_trial/bouncing_model/only_bounce/MATLAB Function ==
  data: t input; states input; u input; angacc_linacc output; FW input; inair_reset_flag input; g parameter; Ixx parameter; Iyy parameter; Izz parameter; m parameter; mf parameter
function angacc_linacc = inair_dynamics(t,states, u, FW, inair_reset_flag, g, Ixx, Iyy, Izz, m, mf)
FG = [0;0;-(mf+6*m)*g];
I_T = [Ixx,0,0;0,Iyy,0;0,0,Izz]; 
r_m1T = [u(1);0;0]; T_v_m1T = [u(7);0;0]; T_a_m1T = [u(13);0;0];
r_m2T = [u(2);0;0]; T_v_m2T = [u(8);0;0]; T_a_m2T = [u(14);0;0];
r_m3T = [0;u(3);0]; T_v_m3T = [0;u(9);0]; T_a_m3T = [0;u(15);0];
r_m4T = [0;u(4);0]; T_v_m4T = [0;u(10);0]; T_a_m4T = [0;u(16);0];
r_m5T = [0;0;u(5)]; T_v_m5T = [0;0;u(11)]; T_a_m5T = [0;0;u(17)];
r_m6T = [0;0;u(6)]; T_v_m6T = [0;0;u(12)]; T_a_m6T = [0;0;u(18)];
r_CMT = m*(r_m1T + r_m2T + r_m3T + r_m4T + r_m5T + r_m6T)/(6*m+mf);
T_v_CMT = m*(T_v_m1T + T_v_m2T + T_v_m3T + T_v_m4T + T_v_m5T + T_v_m6T)/(6*m+mf);
T_a_CMT = m*(T_a_m1T + T_a_m2T + T_a_m3T + T_a_m4T + T_a_m5T + T_a_m6T)/(6*m+mf);
r_CMTx = Vx(r_CMT);r_m1Tx = Vx(r_m1T);r_m2Tx = Vx(r_m2T);r_m3Tx = Vx(r_m3T);
r_m4Tx = Vx(r_m4T);r_m5Tx = Vx(r_m5T);r_m6Tx = Vx(r_m6T);

q0 = states(10); q1 = states(11); q2 = states(12); q3 = states(13);
T_c_O = [q0^2 + q1^2 - q2^2 - q3^2, 2*(q1*q2 + q0*q3), 2*(q1*q3 - q0*q2);...
       2*(q1*q2 - q0*q3), q0^2 - q1^2 + q2^2 - q3^2, 2*(q2*q3 + q0*q1);...
       2*(q1*q3 + q0*q2), 2*(q2*q3 - q0*q1), q0^2 - q1^2 - q2^2 + q3^2];
O_c_T = T_c_O.';

O_v_TO = [states(4);states(5);states(6)];
O_w_T = [states(1);states(2);states(3)];
O_w_Tx = Vx(O_w_T);

C11 =  I_T - m*r_m1Tx*r_m1Tx - m*r_m2Tx*r_m2Tx - m*r_m3Tx*r_m3Tx - m*r_m4Tx*r_m4Tx - m*r_m5Tx*r_m5Tx - m*r_m6Tx*r_m6Tx;
C12 = (mf + 6*m)*r_CMTx*T_c_O;
C21 = -(mf + 6*m)*O_c_T*r_CMTx;
C22 = (mf + 6*m)*eye(3);
D1 = r_CMTx*T_c_O*FG - O_w_Tx*I_T*O_w_T - m*cross(r_m1T,2*O_w_Tx*T_v_m1T + O_w_Tx*O_w_Tx*r_m1T)...
       - m*r_m2Tx*(T_a_m2T + 2*O_w_Tx*T_v_m2T + O_w_Tx*O_w_Tx*r_m2T)...
       - m*r_m3Tx*(T_a_m3T + 2*O_w_Tx*T_v_m3T + O_w_Tx*O_w_Tx*r_m3T)...
       - m*r_m4Tx*(T_a_m4T + 2*O_w_Tx*T_v_m4T + O_w_Tx*O_w_Tx*r_m4T)...
       - m*r_m5Tx*(T_a_m5T + 2*O_w_Tx*T_v_m5T + O_w_Tx*O_w_Tx*r_m5T)...
       - m*r_m6Tx*(T_a_m6T + 2*O_w_Tx*T_v_m6T + O_w_Tx*O_w_Tx*r_m6T);
D2 = FG + FW - (mf + 6*m)*O_c_T*(T_a_CMT + 2*O_w_Tx*T_v_CMT + O_w_Tx*O_w_Tx*r_CMT);
C = [C11,C12;C21,C22]; D = [D1;D2];
OalT_OaTO = C\D;
O_al_T = OalT_OaTO(1:3,1);
O_a_TO = OalT_OaTO(4:6,1);
angacc_linacc = [O_al_T;O_a_TO];
end

== matlab function comprehensive_model_with_rocks_trial/bouncing_model/only_bounce/MATLAB Function4 ==
  data: states input; q_dot output; YY parameter
function q_dot = quaternions_processor(states, YY)

q0 = states(10); q1 = states(11); q2 = states(12); q3 = states(13);
% T_c_O = [q0^2 + q1^2 - q2^2 - q3^2, 2*(q1*q2 + q0*q3), 2*(q1*q3 - q0*q2);...
%        2*(q1*q2 - q0*q3), q0^2 - q1^2 + q2^2 - q3^2, 2*(q2*q3 + q0*q1);...
%        2*(q1*q3 + q0*q2), 2*(q2*q3 - q0*q1), q0^2 - q1^2 - q2^2 + q3^2];
% O_c_T = T_c_O';
% T_c_A = T_c_O*O_c_A;
% A_w_T = [y(1);y(2);y(3)];
% O_w_T = T_c_A*O_w_A + A_w_T;
% wx = O_w_T(1); 
% wy = O_w_T(2);
% wz = O_w_T(3);
wx = states(1); wy = states(2); wz = states(3);
q_dot = ...
      1/2*[0,-wx,-wy,-wz; wx,0,wz,-wy; wy,-wz,0,wx; ...
      wz,wy,-wx,0]*[q0;q1;q2;q3]+YY/2*(1 - [q0,q1,q2,q3]*...
      [q0;q1;q2;q3])*[q0;q1;q2;q3];
end

== matlab function comprehensive_model_with_rocks_trial/bouncing_model1/only_bounce/MATLAB Function2 ==
  data: t input; states input; u input; r_AO input; constraint_flag input; states output; FN input; inair_flag output; par_diffs input; jAp input; surf_numch input; surf_nump input; roll_reset_flag output; inair_reset_flag output; rest_coeff parameter; m parameter; mf parameter; Ixx parameter; R parameter; jA output; must parameter; muk parameter; FN output; surf_num output; Iyy parameter; Izz parameter
function [states, inair_flag, roll_reset_flag, inair_reset_flag, jA, FN, surf_num] = collision_state_set(t,states, u,r_AO, constraint_flag, FN, par_diffs, jAp, surf_numch, surf_nump, rest_coeff, m, mf, Ixx, R, must, muk, Iyy, Izz)
%u1 u2 u3 u4 u5 u6 S1 S2 S3
surf_num = surf_nump;
roll_reset_flag = 0;
inair_reset_flag = 0;
O_w_T = [states(1);states(2);states(3)];
O_v_TO = [states(4);states(5);states(6)];
r_TO = [states(7);states(8);states(9)];
q = [states(10);states(11);states(12);states(13)];
q0 = q(1); q1 = q(2); q2 = q(3); q3 = q(4);

        fx = par_diffs(1,1); 
        fy = par_diffs(2,1);
        fz = par_diffs(3,1);
        kO = [0;0;1];
        iO = [1;0;0];
        jO = [0;1;0];

        if(abs(fx)<=1e-10 && abs(fy)<=1e-10)
            kA = kO;
            jA = jO;
            iA = iO;
            O_c_A = eye(3);
            A_c_O = eye(3);
            flag = 1;
        else
        kA = [fx;fy;fz]/norm([fx;fy;fz]);
        jA = cross(kO,kA)/norm(cross(kO,kA));
        flag = 1;
        if((jAp.')*(jA) < 0)
            jA = -jA;
            flag = 2;
        end
        iA = cross(jA,kA);
        A_c_O = [iA'*iO, iA'*jO, iA'*kO; jA'*iO, jA'*jO, jA'*kO; kA'*iO, kA'*jO, kA'*kO];
        O_c_A = transpose(A_c_O);
        end
O_v_TOa = A_c_O*O_v_TO;        
        
if mod(t,0.001) == 0
if constraint_flag == 0
    inair_flag = true;
 elseif constraint_flag == 1 && FN == 0
             inair_flag = false;
            roll_reset_flag = 1;
            r_TO = r_AO + R*kA;
            surf_num = 0;
elseif constraint_flag == 1 && O_v_TOa(3) >= 0.0001
    inair_flag = true;    
else 
 %%collision response
     
        T_c_O = [q0^2 + q1^2 - q2^2 - q3^2, 2*(q1*q2 + q0*q3), 2*(q1*q3 - q0*q2);...
        2*(q1*q2 - q0*q3), q0^2 - q1^2 + q2^2 - q3^2, 2*(q2*q3 + q0*q1);...
        2*(q1*q3 + q0*q2), 2*(q2*q3 - q0*q1), q0^2 - q1^2 - q2^2 + q3^2];
        O_c_T = T_c_O.';
       
        
        
        T_c_A = T_c_O*O_c_A;
        A_c_T = T_c_A.';
        
        
        l1 = u(1); l2 = u(2); l3 = u(3); l4 = u(4); l5 = u(5); l6 = u(6);
        L33 = Ixx + m*(l3^2 + l4^2 + l5^2 + l6^2);
        L11 = Iyy + m*(l1^2 + l2^2 + l5^2 + l6^2);
        L22 = Izz + m*(l3^2 + l4^2 + l1^2 + l2^2);
        L = A_c_T*[L33,0,0;0,L11,0;0,0,L22]*T_c_A;
        L11 = L(2,2);
        L22 = L(3,3);
        L33 = L(1,1);
        
        mT = mf +6*m;

        w = A_c_T*(O_w_T);
        v = A_c_O*O_v_TO;

        u3 = w(1,1);
        u2 = w(3,1);
        u1 = w(2,1);

        u6 = v(1,1);
        u5 = v(3,1);
        u4 = v(2,1);


        u5_n = -rest_coeff*u5;  
        if abs(u5_n) <= 0.005 %&& FN > 0
            u5_n = 0;
            inair_flag = false;
            roll_reset_flag = 1;
            surf_num = surf_numch;
            r_TO = r_AO + R*kA;
%         elseif abs(u5_n) <= 0.005 && FN < 0
%             u5_n = 0;
%             inair_flag = true;
%             r_TO = r_AO + R*kA;   
        else
            inair_flag = true;
            inair_reset_flag = 1;
             r_TO = r_AO + R*kA;
             FN = 100;
        end
        u2_n = u2;
        u3_n = (L33*u3 - mT*R*u4)/(mT*R^2 + L33);
        u4_n = -R*u3_n;
        u1_n = (L11*u1 + mT*R*u6)/(mT*R^2 + L11);
        u6_n = R*u1_n;
        S1 = mT*(u4_n - u4);
        S2 = mT*(u5_n - u5);
        S3 = mT*(u6_n - u6);

        if ~(sqrt(S1^2 + S3^2) < must*norm(S2))
            alpha = u4 + R*u3;
            gamma = u6 - R*u1;
            k1 = 1/mT + R^2/L11;
            k3 = 1/mT + R^2/L33;
            
            if abs(alpha) > 0
                S1 = S1solve(S2, muk,alpha, gamma, k1, k3); 
                S3 = gamma*S1/(alpha + (k3 - k1)*S1);
                u1_n = u1 - R*S3/L11;
                u3_n = u3 + R*S1/L33;
                u4_n = u4 + S1/mT;
                u6_n = u6 + S3/mT;
            else 
                S3 = S1solve(S2, muk, gamma, alpha, k3, k1);
                S1 = alpha*S3/(gamma + (k1 - k3)*S3);
                u1_n = u1 - R*S3/L11;
                u3_n = u3 + R*S1/L33;
                u4_n = u4 + S1/mT;
                u6_n = u6 + S3/mT;
            end
            
        end

        O_w_T = T_c_A*[u3_n;u1_n;u2_n];
        O_v_TO = O_c_A*[u6_n; u4_n; u5_n];
end
else
    if  constraint_flag == 0
        inair_flag = true;
    else
        inair_flag = false;
    end
end

states = [O_w_T;O_v_TO;r_TO;q];
end

== matlab function comprehensive_model_with_rocks_trial/bouncing_model/onsurface_model/MATLAB Function ==
  data: states input; slip_flag0 output; O_c_A input; R parameter
function slip_flag0 = roll_slip_check(states, O_c_A, R)

q0 = states(10); q1 = states(11); q2 = states(12); q3 = states(13);
T_c_O = [q0^2 + q1^2 - q2^2 - q3^2, 2*(q1*q2 + q0*q3), 2*(q1*q3 - q0*q2);...
       2*(q1*q2 - q0*q3), q0^2 - q1^2 + q2^2 - q3^2, 2*(q2*q3 + q0*q1);...
       2*(q1*q3 + q0*q2), 2*(q2*q3 - q0*q1), q0^2 - q1^2 - q2^2 + q3^2];
O_c_T = T_c_O.';

T_c_A = T_c_O*O_c_A;
A_c_O = O_c_A.';
A_c_T = T_c_A.';

O_v_TO = A_c_O*states(4:6,1);
O_w_T = A_c_T*states(1:3,1);
r_TA =[0;0;R];
OwT_x_rTA = cross(O_w_T, r_TA); 
if abs(O_v_TO(1) - OwT_x_rTA(1)) <= 0.001 && abs(O_v_TO(2) - OwT_x_rTA(2)) <= 0.001
    slip_flag0 = false;
else
    slip_flag0 = true;
end

end

== matlab function comprehensive_model_with_rocks_trial/bouncing_model/onsurface_model/MATLAB Function1 ==
  data: t input; r_AO input; r_AO0 input; roll_reset_flag input; O_v_AO input; O_c_A output; r_TO output; O_w_A output; jA output; par_diffs input; jAp input; flag output; R parameter
function [O_c_A, r_TO,  O_w_A, jA, flag] = calc_OcA_OwA(t, r_AO,r_AO0,roll_reset_flag,O_v_AO, par_diffs, jAp, R)
%change this everytime u change the function
if roll_reset_flag == 1
    r_AO = r_AO0;
end
x_c = r_AO(1);
y_c = r_AO(2);
z_c = r_AO(3);

x_dot = O_v_AO(1);
y_dot = O_v_AO(2);
z_dot = O_v_AO(3);

kO = [0;0;1];
jO = [0;1;0];
iO = [1;0;0];

%z - cos(x/4)-1 = 0;
%- x^2 - y^2 = 0;


fx = par_diffs(1);
fy = par_diffs(2);
fz = par_diffs(3);
fxx = par_diffs(4);
fxy = par_diffs(5);
fxz = par_diffs(6);
fyy = par_diffs(7);
fyz = par_diffs(8);
fzz = par_diffs(9);
fxxx = par_diffs(10);
fxxy = par_diffs(11);
fxxz = par_diffs(12);
fxyy = par_diffs(13);
fxyz = par_diffs(14);
fxzz = par_diffs(15);
fyyy = par_diffs(16);
fyyz = par_diffs(17);
fyzz = par_diffs(18);
fzzz = par_diffs(19);


if(abs(fx)<=1e-20 && abs(fy) <= 1e-20)
    kA = kO;
    jA = jO;
    O_c_A = eye(3);
    A_c_O = eye(3);
    flag = 1;
else
    kA = [fx;fy;fz]/norm([fx;fy;fz]);
    jA = cross(kO,kA)/norm(cross(kO,kA));
    flag = 1;
    if((jAp.')*(jA) < 0)
        jA = -jA;
        flag = 2;
    end
    iA = cross(jA,kA);
    A_c_O = [iA'*iO, iA'*jO, iA'*kO; jA'*iO, jA'*jO, jA'*kO; kA'*iO, kA'*jO, kA'*kO];
    O_c_A = transpose(A_c_O);
end
if flag == 1
    O_w_A = ...
    [-(fx*fxy*x_dot - fy*fxx*x_dot + fx*fyy*y_dot - fy*fxy*y_dot + fx*fyz*z_dot - fy*fxz*z_dot)/((fx^2 + fy^2)^(1/2)*(fx^2 + fy^2 + fz^2)^(1/2));...
     -(fx^2*fxz*x_dot + fy^2*fxz*x_dot + fx^2*fyz*y_dot + fy^2*fyz*y_dot + fx^2*fzz*z_dot + fy^2*fzz*z_dot - fx*fxx*fz*x_dot - fy*fz*fxy*x_dot - fx*fz*fxy*y_dot - fy*fz*fyy*y_dot - fx*fz*fxz*z_dot - fy*fz*fyz*z_dot)/((fx^2 + fy^2)^(1/2)*(fx^2 + fy^2 + fz^2));...
     (fz*(fx*fxy*x_dot - fy*fxx*x_dot + fx*fyy*y_dot - fy*fxy*y_dot + fx*fyz*z_dot - fy*fxz*z_dot))/((fx^2 + fy^2)*(fx^2 + fy^2 + fz^2)^(1/2))];
else
    O_w_A = ...
    [(fx*fxy*x_dot - fy*fxx*x_dot + fx*fyy*y_dot - fy*fxy*y_dot + fx*fyz*z_dot - fy*fxz*z_dot)/((fx^2 + fy^2)^(1/2)*(fx^2 + fy^2 + fz^2)^(1/2));...
     (fx^2*fxz*x_dot + fy^2*fxz*x_dot + fx^2*fyz*y_dot + fy^2*fyz*y_dot + fx^2*fzz*z_dot + fy^2*fzz*z_dot - fx*fxx*fz*x_dot - fy*fz*fxy*x_dot - fx*fz*fxy*y_dot - fy*fz*fyy*y_dot - fx*fz*fxz*z_dot - fy*fz*fyz*z_dot)/((fx^2 + fy^2)^(1/2)*(fx^2 + fy^2 + fz^2));...
     (fz*(fx*fxy*x_dot - fy*fxx*x_dot + fx*fyy*y_dot - fy*fxy*y_dot + fx*fyz*z_dot - fy*fxz*z_dot))/((fx^2 + fy^2)*(fx^2 + fy^2 + fz^2)^(1/2))];
end
if (abs(fx) <= 1e-20 && abs(fy) <= 1e-20)
    O_w_A = [0;0;0];
end
r_TO = r_AO + R*kA;
end

== matlab function comprehensive_model_with_rocks_trial/bouncing_model/onsurface_model/MATLAB Function4 ==
  data: states input; q_dot output; YY parameter
function q_dot = quaternions_processor(states, YY)

q0 = states(10); q1 = states(11); q2 = states(12); q3 = states(13);
% T_c_O = [q0^2 + q1^2 - q2^2 - q3^2, 2*(q1*q2 + q0*q3), 2*(q1*q3 - q0*q2);...
%        2*(q1*q2 - q0*q3), q0^2 - q1^2 + q2^2 - q3^2, 2*(q2*q3 + q0*q1);...
%        2*(q1*q3 + q0*q2), 2*(q2*q3 - q0*q1), q0^2 - q1^2 - q2^2 + q3^2];
% O_c_T = T_c_O';
% T_c_A = T_c_O*O_c_A;
% A_w_T = [y(1);y(2);y(3)];
% O_w_T = T_c_A*O_w_A + A_w_T;
% wx = O_w_T(1); 
% wy = O_w_T(2);
% wz = O_w_T(3);
wx = states(1); wy = states(2); wz = states(3);
q_dot = ...
      1/2*[0,-wx,-wy,-wz; wx,0,wz,-wy; wy,-wz,0,wx; ...
      wz,wy,-wx,0]*[q0;q1;q2;q3]+YY/2*(1 - [q0,q1,q2,q3]*...
      [q0;q1;q2;q3])*[q0;q1;q2;q3];
end
